simulink model "SingleFan"  (R2015b)
settings: Solver=VariableStepAuto  StartTime=1  StopTime=10.0  RelTol=1e-3
libraries: xbsIndex_r4 x22
settings Model: Creator=Stella Modyanto  LastModifiedBy=u228
settings DataIOCC: LimitDataPoints=off
settings DebuggingCC: AllowSymbolicDim=on
settings ModelReferenceCC: PropagateSignalLabelsOutOfModel=on
settings GRTTargetCC: GeneratePreprocessorConditionals=Disable all

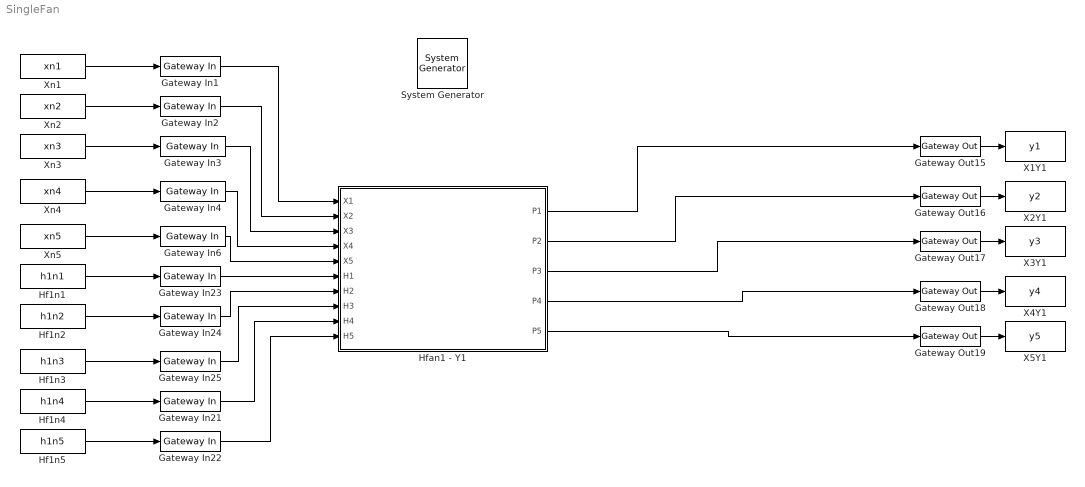
== system SingleFan ==
  " System Generator" : xbsIndex_r4/ System Generator  Tag=genX  xilinxfamily=virtex7  part=xc7vx485t  speed=-2  package=ffg1761  synthesis_tool=Vivado  clock_wrapper=Clock Enables  directory=./netlist  proj_type=Vivado  Synth_file=Vivado Synthesis Defaults  Impl_file=Vivado Implementation Defaults  testbench=off  simulink_period=1  sysclk_period=10  dcm_input_clock_period=10  incr_netlist=off  trim_vbits=Everywhere in SubSystem  dbl_ovrd=According to Block Masks  core_generation=According to Block Masks  run_coregen=off  deprecated_control=off  eval_field=0  block_type=sysgen
  Gateway In{1..4,6,21..25} (10 alike) : xbsIndex_r4/Gateway In  gui_display_data_type=Fixed-point  arith_type="Signed  (2's comp)"  n_bits=16  bin_pt=14  preci_type=Single  exp_width=8  frac_width=24  rows=1  columns=1  quantization="Round  (unbiased: +/- Inf)"  overflow=Saturate  period=1  UseAsADC=off  ADCChannel='1'  interface=None  automatic_assignment=on  address_offset=hex2dec('00')  intf_name=''  intf_description=''  default_value=0  timing_constraint=None  locs_specified=off  LOCs={}  io_standard={}  inherit_from_input=off  hdl_port=on  dbl_ovrd=off  block_type=gatewayin
  Gateway Out{15..19} (5 alike) : xbsIndex_r4/Gateway Out  inherit_from_input=off  hdl_port=on  rows=1  columns=1  UseAsDAC=off  DACChannel='1'  interface=None  automatic_assignment=on  address_offset=hex2dec('00')  intf_name=''  intf_description=''  timing_constraint=None  locs_specified=off  LOCs={}  io_standard={}  block_type=gatewayout
  Hf1n1 : FromWorkspace  VariableName=h1n1  SampleTime=0  OutputAfterFinalValue=Setting to zero
  Hf1n2 : FromWorkspace  VariableName=h1n2  SampleTime=0  OutputAfterFinalValue=Setting to zero
  Hf1n3 : FromWorkspace  VariableName=h1n3  SampleTime=0  OutputAfterFinalValue=Setting to zero
  Hf1n4 : FromWorkspace  VariableName=h1n4  SampleTime=0  OutputAfterFinalValue=Setting to zero
  Hf1n5 : FromWorkspace  VariableName=h1n5  SampleTime=0  OutputAfterFinalValue=Setting to zero
  Hfan1 - Y1 : Subsystem
  X1Y1 : ToWorkspace  VariableName=y1  SampleTime=-1
  X2Y1 : ToWorkspace  VariableName=y2  SampleTime=-1
  X3Y1 : ToWorkspace  VariableName=y3  SampleTime=-1
  X4Y1 : ToWorkspace  VariableName=y4  SampleTime=-1
  X5Y1 : ToWorkspace  VariableName=y5  SampleTime=-1
  "Xn1 " : FromWorkspace  VariableName=xn1  SampleTime=0  OutputAfterFinalValue=Setting to zero
  Xn2 : FromWorkspace  VariableName=xn2  SampleTime=0  OutputAfterFinalValue=Setting to zero
  "Xn3 " : FromWorkspace  VariableName=xn3  SampleTime=0  OutputAfterFinalValue=Setting to zero
  "Xn4 " : FromWorkspace  VariableName=xn4  SampleTime=0  OutputAfterFinalValue=Setting to zero
  Xn5 : FromWorkspace  VariableName=xn5  SampleTime=0  OutputAfterFinalValue=Setting to zero
  wires:
  "Xn1 "/1 -> Gateway In1/1
  Xn2/1 -> Gateway In2/1
  "Xn3 "/1 -> Gateway In3/1
  "Xn4 "/1 -> Gateway In4/1
  Xn5/1 -> Gateway In6/1
  Hf1n1/1 -> Gateway In23/1
  Hf1n2/1 -> Gateway In24/1
  Hf1n3/1 -> Gateway In25/1
  Hf1n4/1 -> Gateway In21/1
  Hf1n5/1 -> Gateway In22/1
  Gateway In1/1 -> Hfan1 - Y1/1(X1)
  Gateway In2/1 -> Hfan1 - Y1/2(X2)
  Gateway In3/1 -> Hfan1 - Y1/3(X3)
  Gateway In4/1 -> Hfan1 - Y1/4(X4)
  Gateway In6/1 -> Hfan1 - Y1/5(X5)
  Gateway In23/1 -> Hfan1 - Y1/6(H1)
  Gateway In24/1 -> Hfan1 - Y1/7(H2)
  Gateway In25/1 -> Hfan1 - Y1/8(H3)
  Gateway In21/1 -> Hfan1 - Y1/9(H4)
  Gateway In22/1 -> Hfan1 - Y1/10(H5)
  Gateway Out15/1 -> X1Y1/1
  Gateway Out19/1 -> X5Y1/1
  Gateway Out18/1 -> X4Y1/1
  Gateway Out17/1 -> X3Y1/1
  Gateway Out16/1 -> X2Y1/1
  Hfan1 - Y1/5(P5) -> Gateway Out19/1
  Hfan1 - Y1/4(P4) -> Gateway Out18/1
  Hfan1 - Y1/3(P3) -> Gateway Out17/1
  Hfan1 - Y1/2(P2) -> Gateway Out16/1
  Hfan1 - Y1/1(P1) -> Gateway Out15/1

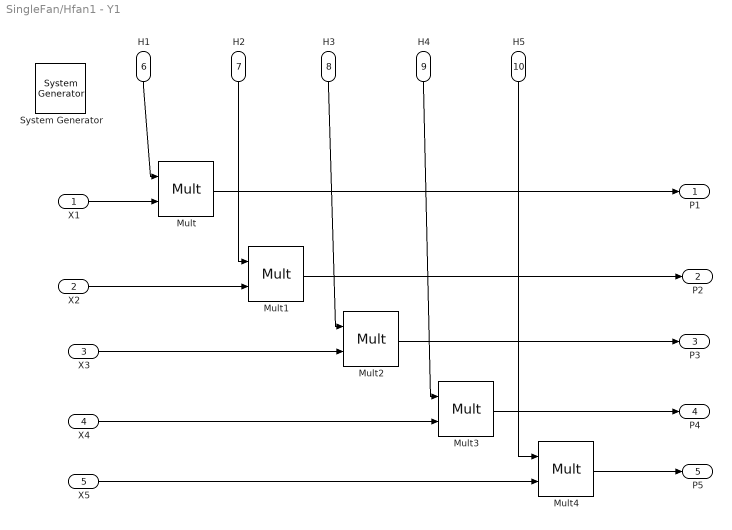
== system SingleFan/Hfan1 - Y1 ==
  X1 : Inport
  X2 : Inport  Port=2
  X3 : Inport  Port=3
  X4 : Inport  Port=4
  X5 : Inport  Port=5
  H1 : Inport  Port=6
  H2 : Inport  Port=7
  H3 : Inport  Port=8
  H4 : Inport  Port=9
  H5 : Inport  Port=10
  " System Generator" : xbsIndex_r4/ System Generator  Tag=genX  xilinxfamily=virtex7  part=xc7vx485t  speed=-2  package=ffg1761  synthesis_tool=Vivado  clock_wrapper=Clock Enables  directory=./netlist  proj_type=Vivado  Synth_file=Vivado Synthesis Defaults  Impl_file=Vivado Implementation Defaults  testbench=off  simulink_period=1  sysclk_period=10  dcm_input_clock_period=10  incr_netlist=off  trim_vbits=Everywhere in SubSystem  dbl_ovrd=According to Block Masks  core_generation=According to Block Masks  run_coregen=off  deprecated_control=off  eval_field=0  block_type=sysgen
  Mult{,1..4} (5 alike) : xbsIndex_r4/Mult  precision=Full  arith_type="Signed  (2's comp)"  n_bits=16  bin_pt=14  quantization=Truncate  overflow=Wrap  en=off  latency=3  use_behavioral_HDL=off  opt=Speed  use_embedded=on  optimum_pipeline=off  pipeline=on  dbl_ovrd=off  use_rpm=on  placement_style=Triangular  block_type=mult
  P1 : Outport
  P2 : Outport  Port=2
  P3 : Outport  Port=3
  P4 : Outport  Port=4
  P5 : Outport  Port=5
  wires:
  Mult/1 -> P1/1
  Mult1/1 -> P2/1
  Mult4/1 -> P5/1
  Mult2/1 -> P3/1
  Mult3/1 -> P4/1
  X1/1 -> Mult/2
  H1/1 -> Mult/1
  H2/1 -> Mult1/1
  X2/1 -> Mult1/2
  X3/1 -> Mult2/2
  H3/1 -> Mult2/1
  H4/1 -> Mult3/1
  X4/1 -> Mult3/2
  X5/1 -> Mult4/2
  H5/1 -> Mult4/1
